simulink model "EV3_test"  (Simulink 9.0)
settings: Solver=FixedStepDiscrete  StartTime=0.0  StopTime=Inf  RelTol=1e-3  EnableMultiTasking=on
values from neighbouring files (symbols this model uses):
  K = acker(s1z.a, s1z.b, [0.2225 0.9743 0.987 0.987])    [model.m]
  K_PWM = 8.087    [model.m]
  l = 0.125    [model.m]
  R = 0.027    [model.m]
  Ts = 0.0033    [model.m]
undefined symbols (not defined in the file or in its folder): DiscIntNeverNeededParam
libraries: simulink x3, rpi_blkst x1
settings Model: Creator=jacques  LastModifiedBy=USER  SimulationMode=external
settings DataIOCC: LimitDataPoints=on  SignalLoggingSaveFormat=ModelDataLogs
settings OptimizationCC: ExpressionDepthLimit=2147483647  LifeSpan=1
settings DebuggingCC: SolverPrmCheckMsg=warning  FcnCallInpInsideContextMsg=warning  StateNameClashWarn=warning
settings HardwareCC: ProdLargestAtomicInteger=Long  ProdLargestAtomicFloat=Double  ProdIntDivRoundTo=Zero  ProdEndianess=LittleEndian  ProdHWDeviceType=ARM Compatible->ARM 11
settings SFSimCC: MATLABDynamicMemAlloc=off
settings RTWCC: SystemTargetFile=ert_rpi.tlc  TemplateMakefile=ert_rpi.tmf  PostCodeGenCommand=postGenFunc(buildInfo)  Description=RTW Embedded Coder RPI target
settings CodeAppCC: IgnoreCustomStorageClasses=off  CustomSymbolStrType=$N$R$M  InternalIdentifier=Classic
settings STFCustomTargetCC: ModelReferenceCompliant=off  CombineOutputUpdateFcns=on  ERTCustomFileBanners=on  SupportNonInlinedSFcns=off  RemoveResetFunc=on  MATLABClassNameForMDSCustomization=Simulink.SoftwareTarget.ERTCustomization  GRTInterface=off  SystemTargetFile=ert_rpi.tlc
settings ERTTargetCC: MultiwordLength=2048  ModelReferenceCompliant=off  ParMdlRefBuildCompliant=off  CompOptLevelCompliant=off  ConcurrentExecutionCompliant=off  SupportContinuousTime=on  ModelStepFunctionPrototypeControlCompliant=off  CPPClassGenCompliant=off  UseToolchainInfoCompliant=off  ExtMode=on  ExtModeMexArgs='192.168.43.59'  ERTCustomFileTemplate=ert_rpi_file_process.tlc  ConvertIfToSwitch=off  SuppressUnreachableDefaultCases=off

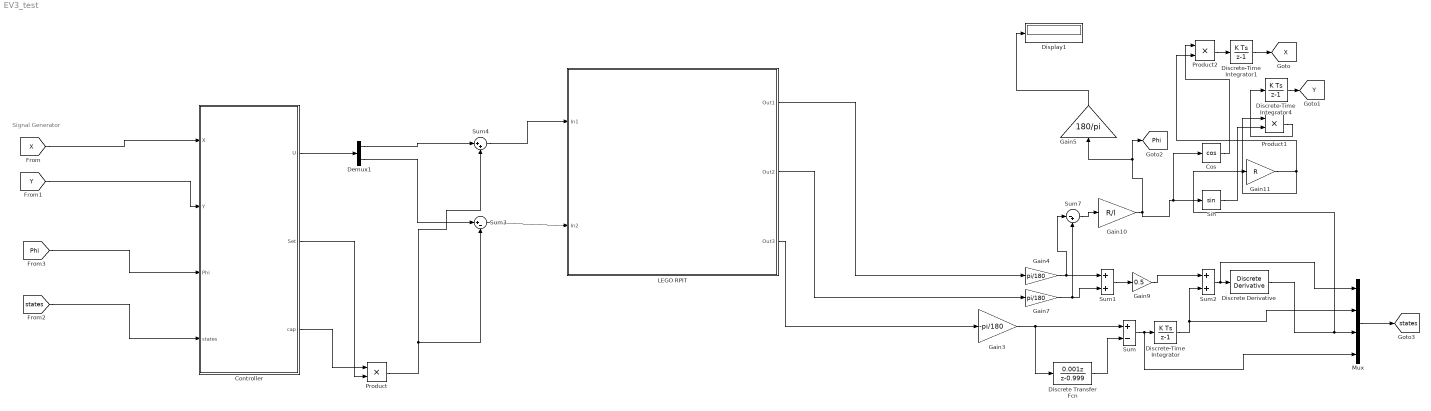
== system EV3_test ==
  note: Signal Generator
  Controller : Stateflow chart  TreatAsAtomicUnit=on
  Cos : Trigonometry  Operator=cos
  Demux1 : Demux  Outputs=2
  Discrete Transfer Fcn : DiscreteTransferFcn  Numerator=[0.001 0]  Denominator=[1 -0.999]  SampleTime=Ts
  Discrete Derivative : simulink/Discrete/Discrete Derivative  gainval=1.0  ICPrevScaledInput=0.0  OutMin=[]  OutMax=[]  OutDataType=fixdt(1, 16)  OutScaling=2^-10  DoSatur=off
  Discrete-Time Integrator : DiscreteIntegrator  InitialConditionSetting=State (most efficient)  SampleTime=Ts  ICPrevOutput=DiscIntNeverNeededParam  ICPrevScaledInput=DiscIntNeverNeededParam
  Discrete-Time Integrator1 : DiscreteIntegrator  InitialConditionSetting=State (most efficient)  SampleTime=Ts  ICPrevOutput=DiscIntNeverNeededParam  ICPrevScaledInput=DiscIntNeverNeededParam
  Discrete-Time Integrator4 : DiscreteIntegrator  InitialConditionSetting=State (most efficient)  SampleTime=Ts  ICPrevOutput=DiscIntNeverNeededParam  ICPrevScaledInput=DiscIntNeverNeededParam
  Display1 : Display
  Gain10 : Gain  Gain=R/l
  Gain11 : Gain  Gain=R
  Gain3 : Gain  Gain=-pi/180
  Gain4 : Gain  Gain=pi/180
  Gain5 : Gain  Gain=180/pi
  Gain7 : Gain  Gain=pi/180
  Gain9 : Gain  Gain=0.5
  "LEGO RPIT " : Subsystem
  Mux : Mux
  Product : Product
  Product1 : Product
  Product2 : Product
  Sin : Trigonometry
  Sum : Sum  Inputs=+-
  Sum1 : Sum
  Sum2 : Sum
  Sum3 : Sum  Inputs=|+-
  Sum4 : Sum  Inputs=|++
  Sum7 : Sum  Inputs=|-+
  tag scope: Phi=global, X=global, Y=global, states=global
  wires:
  Controller/1(U) -> Demux1/1
  Demux1/1 -> Sum4/1
  Demux1/2 -> Sum3/1
  Product/1 -> Sum3/2, Sum4/2
  Controller/2(Set) -> Product/2
  Controller/3(cap) -> Product/1
  [Y] -> Controller/2(Y)
  [states] -> Controller/4(states)
  [X] -> Controller/1(X)
  [Phi] -> Controller/3(Phi)
  Gain7/1 -> Sum7/2, Sum1/2
  Gain3/1 -> Discrete Transfer Fcn/1, Sum/1
  Discrete-Time Integrator/1 -> Mux/2, Sum2/2
  Sum/1 -> Mux/4, Discrete-Time Integrator/1
  Mux/1 -> [states]
  Sum1/1 -> Gain9/1
  Sin/1 -> Product1/2
  Cos/1 -> Product2/1
  Discrete-Time Integrator1/1 -> [X]
  Product1/1 -> Discrete-Time Integrator4/1
  Gain11/1 -> Product1/1, Product2/2
  Sum7/1 -> Gain10/1
  Gain5/1 -> Display1/1
  Discrete-Time Integrator4/1 -> [Y]
  Product2/1 -> Discrete-Time Integrator1/1
  Gain10/1 -> Cos/1, Sin/1, Gain5/1, [Phi]
  Sum2/1 -> Mux/1, Discrete Derivative/1
  Discrete Derivative/1 -> Gain11/1, Mux/3
  Discrete Transfer Fcn/1 -> Sum/2
  Gain4/1 -> Sum7/1, Sum1/1
  Gain9/1 -> Sum2/1
  Sum4/1 -> "LEGO RPIT "/1(In1)
  Sum3/1 -> "LEGO RPIT "/2(In2)
  "LEGO RPIT "/1(Out1) -> Gain4/1
  "LEGO RPIT "/2(Out2) -> Gain7/1
  "LEGO RPIT "/3(Out3) -> Gain3/1

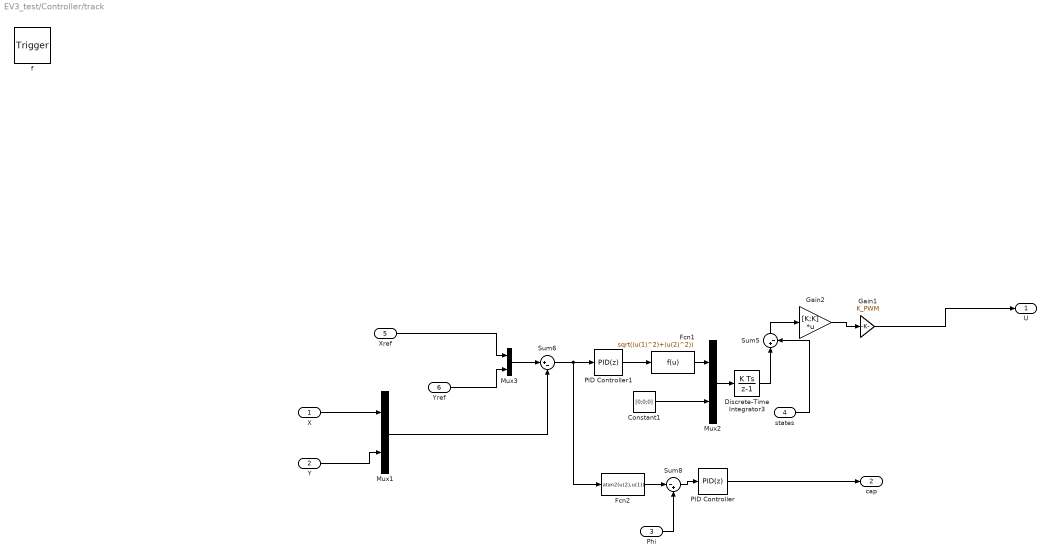
== system EV3_test/Controller/track ==
  X : Inport  OutDataTypeStr=double  PortDimensions=1
  Y : Inport  Port=2  OutDataTypeStr=double  PortDimensions=1
  Phi : Inport  Port=3  OutDataTypeStr=double  PortDimensions=1
  states : Inport  Port=4  OutMin=[4]  OutMax=[4]  OutDataTypeStr=double  PortDimensions=4
  Xref : Inport  Port=5  OutDataTypeStr=double  PortDimensions=1
  Yref : Inport  Port=6  OutDataTypeStr=double  PortDimensions=1
  f : TriggerPort  TriggerType=function-call  VariantControl=(inherit)
      settings: CopyFcn=Stateflow.SLINSF.SimulinkMan.removeBlockPreDeleteFcn  PreDeleteFcn=Stateflow.SLINSF.SimulinkMan.unsafePredeleteFcn
  Constant1 : Constant  Value=[0;0;0]
  Discrete-Time Integrator3 : DiscreteIntegrator  SampleTime=-1  ICPrevOutput=DiscIntNeverNeededParam  ICPrevScaledInput=DiscIntNeverNeededParam
  Fcn1 : Fcn  Expr=sqrt((u(1)^2)+(u(2)^2))
  Fcn2 : Fcn  Expr=atan2(u(2),u(1))
  Gain1 : Gain  Gain=K_PWM
  Gain2 : Gain  Gain=[K;K]  Multiplication=Matrix(K*u)
  Mux1 : Mux  Inputs=2
  Mux2 : Mux  Inputs=2
  Mux3 : Mux  Inputs=2
  PID Controller : simulink/Continuous/PID Controller  Controller=PID  TimeDomain=Discrete-time  SampleTime=-1  IntegratorMethod=Forward Euler  FilterMethod=Forward Euler  Form=Parallel  UseFilter=on  ControllerParametersSource=internal  P=4  I=0  D=0.8  N=100  InitialConditionSource=internal  InitialConditionForIntegrator=0  InitialConditionForFilter=0  ExternalReset=none  LimitOutput=off  UpperSaturationLimit=inf  LowerSaturationLimit=-inf  LinearizeAsGain=on  AntiWindupMode=none  Kb=1  TrackingMode=off  Kt=1  PParamMin=[]  PParamMax=[]  IParamMin=[]  IParamMax=[]  DParamMin=[]  DParamMax=[]  NParamMin=[]  NParamMax=[]  KbParamMin=[]  KbParamMax=[]  KtParamMin=[]  KtParamMax=[]  POutMin=[]  POutMax=[]  IOutMin=[]  IOutMax=[]  DOutMin=[]  DOutMax=[]  NOutMin=[]  NOutMax=[]  KbOutMin=[]  KbOutMax=[]  KtOutMin=[]  KtOutMax=[]  IntegratorOutMin=[]  IntegratorOutMax=[]  FilterOutMin=[]  FilterOutMax=[]  SumOutMin=[]  SumOutMax=[]  SumI1OutMin=[]  SumI1OutMax=[]  SumI2OutMin=[]  SumI2OutMax=[]  SumI3OutMin=[]  SumI3OutMax=[]  SumDOutMin=[]  SumDOutMax=[]  SaturationOutMin=[]  SaturationOutMax=[]  IntegratorContinuousStateAttributes=''  IntegratorStateMustResolveToSignalObject=off  IntegratorRTWStateStorageClass=Auto  FilterContinuousStateAttributes=''  FilterStateMustResolveToSignalObject=off  FilterRTWStateStorageClass=Auto  DifferentiatorICPrevScaledInput=0  DifferentiatorOutMin=[]  DifferentiatorOutMax=[]  InitialConditionSetting=State (most efficient)  FilterDiffOutCoefMin=[]  FilterDiffOutCoefMax=[]  SumDenOutMin=[]  SumDenOutMax=[]  SumNumOutMin=[]  SumNumOutMax=[]  ReciprocalOutMin=[]  ReciprocalOutMax=[]  DivideOutMin=[]  DivideOutMax=[]  TunerSelectOption=Transfer Function Based (PID Tuner App)
  PID Controller1 : simulink/Continuous/PID Controller  Controller=PID  TimeDomain=Discrete-time  SampleTime=-1  IntegratorMethod=Forward Euler  FilterMethod=Forward Euler  Form=Parallel  UseFilter=on  ControllerParametersSource=internal  P=1  I=0.025  D=0.105  N=100  InitialConditionSource=internal  InitialConditionForIntegrator=0  InitialConditionForFilter=0  ExternalReset=none  LimitOutput=off  UpperSaturationLimit=inf  LowerSaturationLimit=-inf  LinearizeAsGain=on  AntiWindupMode=none  Kb=1  TrackingMode=off  Kt=1  PParamMin=[]  PParamMax=[]  IParamMin=[]  IParamMax=[]  DParamMin=[]  DParamMax=[]  NParamMin=[]  NParamMax=[]  KbParamMin=[]  KbParamMax=[]  KtParamMin=[]  KtParamMax=[]  POutMin=[]  POutMax=[]  IOutMin=[]  IOutMax=[]  DOutMin=[]  DOutMax=[]  NOutMin=[]  NOutMax=[]  KbOutMin=[]  KbOutMax=[]  KtOutMin=[]  KtOutMax=[]  IntegratorOutMin=[]  IntegratorOutMax=[]  FilterOutMin=[]  FilterOutMax=[]  SumOutMin=[]  SumOutMax=[]  SumI1OutMin=[]  SumI1OutMax=[]  SumI2OutMin=[]  SumI2OutMax=[]  SumI3OutMin=[]  SumI3OutMax=[]  SumDOutMin=[]  SumDOutMax=[]  SaturationOutMin=[]  SaturationOutMax=[]  IntegratorContinuousStateAttributes=''  IntegratorStateMustResolveToSignalObject=off  IntegratorRTWStateStorageClass=Auto  FilterContinuousStateAttributes=''  FilterStateMustResolveToSignalObject=off  FilterRTWStateStorageClass=Auto  DifferentiatorICPrevScaledInput=0  DifferentiatorOutMin=[]  DifferentiatorOutMax=[]  InitialConditionSetting=State (most efficient)  FilterDiffOutCoefMin=[]  FilterDiffOutCoefMax=[]  SumDenOutMin=[]  SumDenOutMax=[]  SumNumOutMin=[]  SumNumOutMax=[]  ReciprocalOutMin=[]  ReciprocalOutMax=[]  DivideOutMin=[]  DivideOutMax=[]  TunerSelectOption=Transfer Function Based (PID Tuner App)
  Sum5 : Sum  Inputs=|+-
  Sum6 : Sum  Inputs=|+-
  Sum8 : Sum  Inputs=|-+
  U : Outport  InitialOutput=[0;0]
  cap : Outport  Port=2  InitialOutput=[0]
  wires:
  Y/1 -> Mux1/2
  X/1 -> Mux1/1
  Discrete-Time Integrator3/1 -> Sum5/1
  Fcn1/1 -> Mux2/1
  Phi/1 -> Sum8/2
  Xref/1 -> Mux3/1
  Sum5/1 -> Gain2/1
  Yref/1 -> Mux3/2
  Sum8/1 -> PID Controller/1
  Fcn2/1 -> Sum8/1
  Mux2/1 -> Discrete-Time Integrator3/1
  Sum6/1 -> PID Controller1/1, Fcn2/1
  Gain2/1 -> Gain1/1
  PID Controller1/1 -> Fcn1/1
  Mux1/1 -> Sum6/2
  Constant1/1 -> Mux2/2
  Mux3/1 -> Sum6/1
  Gain1/1 -> U/1
  states/1 -> Sum5/2
  PID Controller/1 -> cap/1

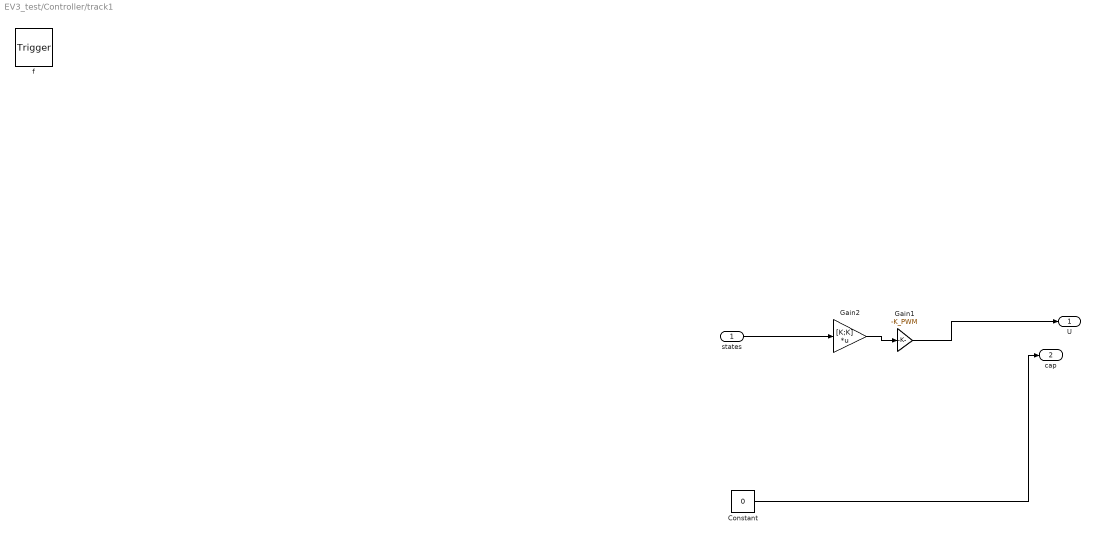
== system EV3_test/Controller/track1 ==
  states : Inport  OutMin=[4]  OutMax=[4]  OutDataTypeStr=double  PortDimensions=4
  f : TriggerPort  TriggerType=function-call  VariantControl=(inherit)
      settings: CopyFcn=Stateflow.SLINSF.SimulinkMan.removeBlockPreDeleteFcn  PreDeleteFcn=Stateflow.SLINSF.SimulinkMan.unsafePredeleteFcn
  Constant : Constant  Value=0
  Gain1 : Gain  Gain=-K_PWM
  Gain2 : Gain  Gain=[K;K]  Multiplication=Matrix(K*u)
  U : Outport  InitialOutput=[0;0]
  cap : Outport  Port=2  InitialOutput=[0]
  wires:
  states/1 -> Gain2/1
  Gain2/1 -> Gain1/1
  Gain1/1 -> U/1
  Constant/1 -> cap/1

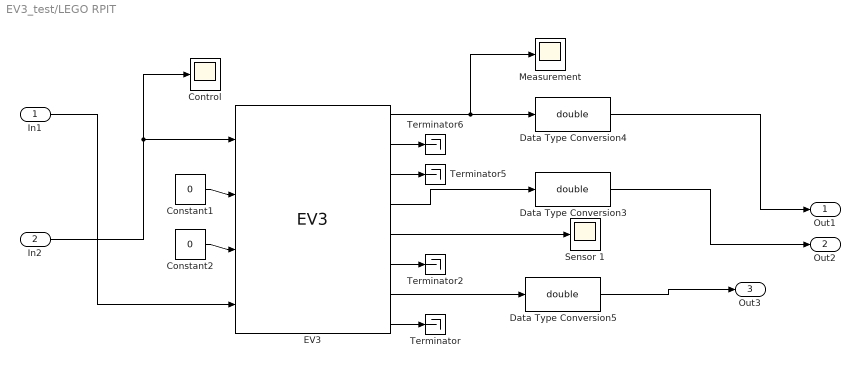
== system EV3_test/LEGO RPIT  ==
  In1 : Inport
  In2 : Inport  Port=2
  Constant1 : Constant  Value=0
  Constant2 : Constant  Value=0
  Control : Scope
  Data Type Conversion3 : DataTypeConversion  OutDataTypeStr=double
  Data Type Conversion4 : DataTypeConversion  OutDataTypeStr=double
  Data Type Conversion5 : DataTypeConversion  OutDataTypeStr=double
  EV3 : rpi_blkst/EV3  rpi_mask_Ts=0.0033
      settings: SourceProductName=RPI Blockset
  Measurement : Scope
  Sensor 1 : Scope
  Terminator{,2,5..6} (4 alike) : Terminator
  Out1 : Outport
  Out2 : Outport  Port=2
  Out3 : Outport  Port=3
  wires:
  Data Type Conversion5/1 -> Out3/1
  EV3/6 -> Terminator2/1
  In1/1 -> EV3/4
  EV3/7 -> Data Type Conversion5/1
  EV3/4 -> Data Type Conversion3/1
  Constant2/1 -> EV3/3
  In2/1 -> Control/1, EV3/1
  Constant1/1 -> EV3/2
  EV3/5 -> Sensor 1/1
  EV3/3 -> Terminator5/1
  EV3/2 -> Terminator6/1
  EV3/1 -> Data Type Conversion4/1, Measurement/1
  EV3/8 -> Terminator/1
  Data Type Conversion3/1 -> Out2/1
  Data Type Conversion4/1 -> Out1/1

== stateflow chart Controller ==
  settings: updateMethod=DISCRETE  sampleTime=0.0033
  state GoToGoal
    entry:
    i=1;
    P=waypoints(:,i);
    Xref=P(1);
    Yref=P(2);
    %Set=0;
    Set=1;
    during:
    % [U,cap]=track1(states);
    [U,cap]= track(X,Y,Phi,states,Xref,Yref);
    V=sqrt(((Xref-X)^2)+((Yref-Y)^2));
  state Track [commented out]
    during:
    [U,cap]= track(X,Y,Phi,states,Xref,Yref),Set=1;
    V=sqrt(((Xref-X)^2)+((Yref-Y)^2));
    exit:
    i=i+1;
  state NextGoal [commented out]
    entry:
    P=waypoints(:,i)
    Xref=P(1);
    Yref=P(2);
    during:
    Set=1;
    [U,cap]= track(X,Y,Phi,states,Xref,Yref);
    V=sqrt(((Xref-X)^2)+((Yref-Y)^2));
    exit:
    i=i+1;
  state Stop
    during:
    Set=0;
    [U,cap]=track1(states);
  state [U,cap] = track(X,Y,Phi,states,Xref,Yref) [function]
  state [U,cap] = track1(states) [function]
  (default) -> GoToGoal
  Stop -> NextGoal [commented out] : [after(2,sec)]
  GoToGoal -> Stop : [V<0.1]{i=i+1;}
  NextGoal -> Stop [commented out] : [V<0.02 ]
  Stop -> Stop [commented out] : [norm(P-waypoints(:,4))==0]
  (default) -> Track [commented out] : [after(3,sec)]
  data: X function_input double size=1; Y function_input double size=1; Phi function_input double size=1; U function_output double; states function_input double size=4; Xref function_input double size=1; Yref function_input double size=1; cap function_output double; U function_output double; states function_input double size=4; cap function_output double; X input double; Y input double; Phi input double; states input double size=[4,1] [4..4]; U output double [4..4]; waypoints parameter double; i local double; P local double; Yref local double; Xref local double; V local double; Set output double; cap output double
